simulink model "electric_motor"  (R2016b)
settings: Solver=FixedStepAuto  StartTime=0.0  StopTime=10.0  FixedStep=0.001  RelTol=1e-3
values from neighbouring files (symbols this model uses):
  b = 0.00513710988005    [exp1234_estimated_parameters.mat]    (also in exp123_estimated_parameters.mat = 0.00708301164632; exp3_estimated_parameters.mat = 0.015214111895; exp3_estimated_parameters2.mat = 0.0114899753562; motor_calculated_parameters.mat = 0.0173555097)
  beta = 0.000873619169313    [exp1234_estimated_parameters.mat]    (also in exp123_estimated_parameters.mat = 0.000840675695047; exp3_estimated_parameters.mat = 0.000887479829086; exp3_estimated_parameters2.mat = 0.000474777840732; motor_calculated_parameters.mat = 0.000149678)
  J = 0.00106248635811    [exp1234_estimated_parameters.mat]    (also in exp123_estimated_parameters.mat = 0.0010108834441; exp3_estimated_parameters.mat = 0.00123090750882; exp3_estimated_parameters2.mat = 0.000928195104658; motor_calculated_parameters.mat = 0.00123078313678)
  R = 2.45072469052    [exp1234_estimated_parameters.mat]    (also in exp123_estimated_parameters.mat; exp3_estimated_parameters.mat = 1.83400285093; exp3_estimated_parameters2.mat; motor_calculated_parameters.mat = 2.39)
undefined symbols (not defined in the file): i_N, omega_N, u_N
settings Model: Creator=piotr  LastModifiedBy=piotr

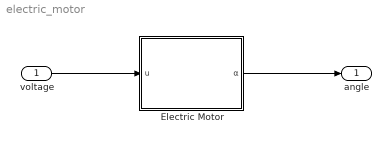
== system electric_motor ==
  voltage : Inport
  Electric Motor : Subsystem  mask{K=(u_N-R*i_N)/omega_N, R=R, beta=beta, b=b, J=J}
      mask prompts: K "Motor constant"; R "Electrical resistance [Ω]"; beta "Motor viscous damping [N*m*s/rad]"; b "Motor dry damping [N*m]"; J "Motor moment of inertia [kg*m^2]"
  angle : Outport
  wires:
  voltage/1 -> Electric Motor/1(u)
  Electric Motor/1(α) -> angle/1

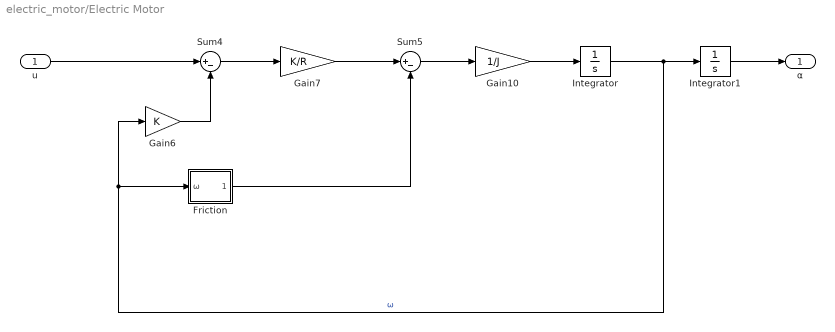
== system electric_motor/Electric Motor ==
  u : Inport
  Friction : Subsystem
  Gain10 : Gain  Gain=1/J
  Gain6 : Gain  Gain=K
  Gain7 : Gain  Gain=K/R
  Integrator : Integrator
  Integrator1 : Integrator
  Sum4 : Sum  Inputs=|+-
  Sum5 : Sum  Inputs=|+-
  α : Outport
  wires:
  Integrator/1 -> Integrator1/1, Gain6/1, Friction/1(ω)  "ω"
  u/1 -> Sum4/1
  Gain6/1 -> Sum4/2
  Sum4/1 -> Gain7/1
  Gain7/1 -> Sum5/1
  Sum5/1 -> Gain10/1
  Gain10/1 -> Integrator/1
  Integrator1/1 -> α/1
  Friction/1(Out1) -> Sum5/2

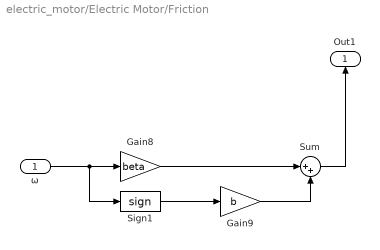
== system electric_motor/Electric Motor/Friction ==
  ω : Inport
  Gain8 : Gain  Gain=beta
  Gain9 : Gain  Gain=b
  Sign1 : Signum  ZeroCross=off
  Sum : Sum  Inputs=|++
  Out1 : Outport
  wires:
  ω/1 -> Sign1/1, Gain8/1
  Sign1/1 -> Gain9/1
  Gain8/1 -> Sum/1
  Sum/1 -> Out1/1
  Gain9/1 -> Sum/2
